simulink model "Input_Output"  (R2016b)
settings: Solver=FixedStepDiscrete  StartTime=0.0  StopTime=inf  FixedStep=InpOutp.tiSimnTiStep_C  RelTol=1e-3  EnableMultiTasking=on
settings Model: Creator=m01wolf  LastModifiedBy=bunver
settings DataIOCC: SaveFormat=StructureWithTime  SaveOutput=off  DSMLogging=off  VisualizeSimOutput=off  SaveTime=off  SignalLoggingName=Results
settings OptimizationCC: BlockReduction=off  ConditionallyExecuteInputs=off  LifeSpan=inf
settings DebuggingCC: AllowSymbolicDim=off  SFUnexpectedBacktrackingDiag=warning  SFNoUnconditionalDefaultTransitionDiag=warning  SFExecutionAtInitializationDiag=none
settings ModelReferenceCC: ModelReferenceNumInstancesAllowed=Single  PropagateSignalLabelsOutOfModel=off
settings GRTTargetCC: TargetLangStandard=C89/C90 (ANSI)
settings ConfigComp: CovMetricSettings=dw  CovHtmlReporting=on  CovSaveCumulativeToWorkspaceVar=on  CovSaveSingleToWorkspaceVar=on  CovExternalEMLEnable=off

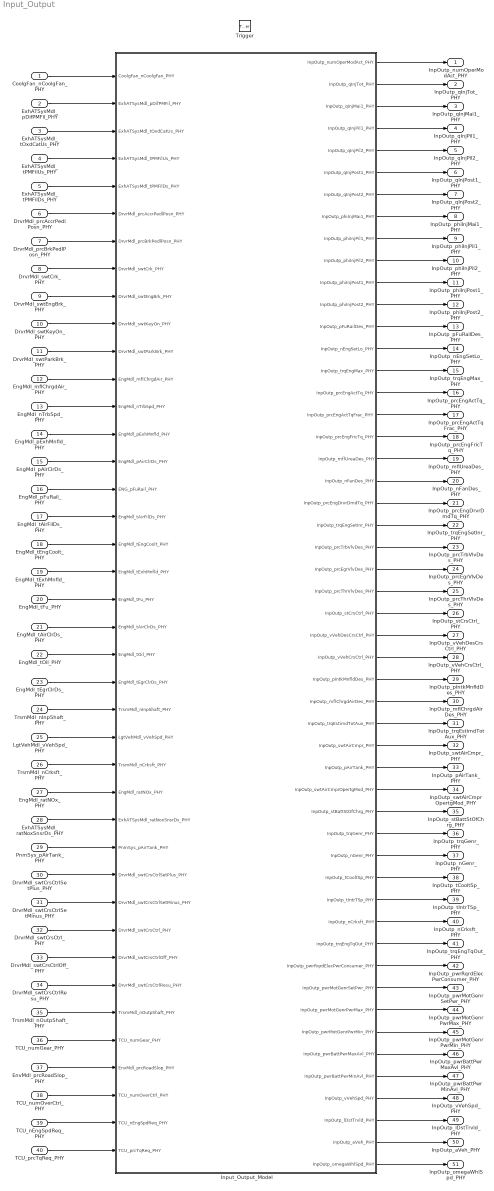
== system Input_Output ==
  CoolgFan_nCoolgFan_PHY : Inport
  ExhATSysMdl_pDifPMFil_PHY : Inport  Port=2
  ExhATSysMdl_tOxdCatUs_PHY : Inport  Port=3
  ExhATSysMdl_tPMFilUs_PHY : Inport  Port=4
  ExhATSysMdl_tPMFilDs_PHY : Inport  Port=5
  DrvrMdl_prcAccrPedlPosn_PHY : Inport  Port=6
  DrvrMdl_prcBrkPedlPosn_PHY : Inport  Port=7
  DrvrMdl_swtCrk_PHY : Inport  Port=8
  DrvrMdl_swtEngBrk_PHY : Inport  Port=9
  DrvrMdl_swtKeyOn_PHY : Inport  Port=10
  DrvrMdl_swtParkBrk_PHY : Inport  Port=11
  EngMdl_mflChrgdAir_PHY : Inport  Port=12
  EngMdl_nTrbSpd_PHY : Inport  Port=13
  EngMdl_pExhMnfld_PHY : Inport  Port=14
  EngMdl_pAirClrDs_PHY : Inport  Port=15
  EngMdl_pFuRail_PHY : Inport  Port=16
  EngMdl_tAirFilDs_PHY : Inport  Port=17
  EngMdl_tEngCoolt_PHY : Inport  Port=18
  EngMdl_tExhMnfld_PHY : Inport  Port=19
  EngMdl_tFu_PHY : Inport  Port=20
  EngMdl_tAirClrDs_PHY : Inport  Port=21
  EngMdl_tOil_PHY : Inport  Port=22
  EngMdl_tEgrClrDs_PHY : Inport  Port=23
  TrsmMdl_nInpShaft_PHY : Inport  Port=24
  LgtVehMdl_vVehSpd_PHY : Inport  Port=25
  TrsmMdl_nCrksft_PHY : Inport  Port=26
  EngMdl_ratNOx_PHY : Inport  Port=27
  ExhATSysMdl_ratNoxSnsrDs_PHY : Inport  Port=28
  PnmSys_pAirTank_PHY : Inport  Port=29
  DrvrMdl_swtCrsCtrlSetPlus_PHY : Inport  Port=30
  DrvrMdl_swtCrsCtrlSetMinus_PHY : Inport  Port=31
  DrvrMdl_swtCrsCtrl_PHY : Inport  Port=32
  DrvrMdl_swtCrsCtrlOff_PHY : Inport  Port=33
  DrvrMdl_swtCrsCtrlResu_PHY : Inport  Port=34
  TrsmMdl_nOutpShaft_PHY : Inport  Port=35
  TCU_numGear_PHY : Inport  Port=36
  EnvMdl_prcRoadSlop_PHY : Inport  Port=37
  TCU_numOverCtrl_PHY : Inport  Port=38
  TCU_nEngSpdReq_PHY : Inport  Port=39
  TCU_prcTqReq_PHY : Inport  Port=40
  Trigger : TriggerPort  TriggerType=function-call  VariantControl=Variant  PortDimensions=1
  Input_Output_Model : Subsystem
  InpOutp_numOperModAct_PHY : Outport
  InpOutp_qInjTot_PHY : Outport  Port=2
  InpOutp_qInjMai1_PHY : Outport  Port=3
  InpOutp_qInjPil1_PHY : Outport  Port=4
  InpOutp_qInjPil2_PHY : Outport  Port=5
  InpOutp_qInjPost1_PHY : Outport  Port=6
  InpOutp_qInjPost2_PHY : Outport  Port=7
  InpOutp_phiInjMai1_PHY : Outport  Port=8
  InpOutp_phiInjPil1_PHY : Outport  Port=9
  InpOutp_phiInjPil2_PHY : Outport  Port=10
  InpOutp_phiInjPost1_PHY : Outport  Port=11
  InpOutp_phiInjPost2_PHY : Outport  Port=12
  InpOutp_pFuRailDes_PHY : Outport  Port=13
  InpOutp_nEngSetLo_PHY : Outport  Port=14
  InpOutp_trqEngMax_PHY : Outport  Port=15
  InpOutp_prcEngActTq_PHY : Outport  Port=16
  InpOutp_prcEngActTqFrac_PHY : Outport  Port=17
  InpOutp_prcEngFricTq_PHY : Outport  Port=18
  InpOutp_mflUreaDes_PHY : Outport  Port=19
  InpOutp_nFanDes_PHY : Outport  Port=20
  InpOutp_prcEngDrvrDmdTq_PHY : Outport  Port=21
  InpOutp_trqEngSetInr_PHY : Outport  Port=22
  InpOutp_prcTrbVlvDes_PHY : Outport  Port=23
  InpOutp_prcEgrVlvDes_PHY : Outport  Port=24
  InpOutp_prcThrVlvDes_PHY : Outport  Port=25
  InpOutp_stCrsCtrl_PHY : Outport  Port=26
  InpOutp_vVehDesCrsCtrl_PHY : Outport  Port=27
  InpOutp_vVehCrsCtrl_PHY : Outport  Port=28
  InpOutp_pIntkMnfldDes_PHY : Outport  Port=29
  InpOutp_mflChrgdAirDes_PHY : Outport  Port=30
  InpOutp_trqEstimdTotAux_PHY : Outport  Port=31
  InpOutp_swtAirCmpr_PHY : Outport  Port=32
  InpOutp_pAirTank_PHY : Outport  Port=33
  InpOutp_swtAirCmprOpertgMod_PHY : Outport  Port=34
  InpOutp_stBattStOfChrg_PHY : Outport  Port=35
  InpOutp_trqGenr_PHY : Outport  Port=36
  InpOutp_nGenr_PHY : Outport  Port=37
  InpOutp_tCooltSp_PHY : Outport  Port=38
  InpOutp_tIntrTSp_PHY : Outport  Port=39
  InpOutp_nCrksft_PHY : Outport  Port=40
  InpOutp_trqEngTqOut_PHY : Outport  Port=41
  InpOutp_pwrRqrdElecPwrConsumer_PHY : Outport  Port=42
  InpOutp_pwrMotGenrSetPwr_PHY : Outport  Port=43
  InpOutp_pwrMotGenrPwrMax_PHY : Outport  Port=44
  InpOutp_pwrMotGenrPwrMin_PHY : Outport  Port=45
  InpOutp_pwrBattPwrMaxAvl_PHY : Outport  Port=46
  InpOutp_pwrBattPwrMinAvl_PHY : Outport  Port=47
  InpOutp_vVehSpd_PHY : Outport  Port=48
  InpOutp_lDstTrvld_PHY : Outport  Port=49
  InpOutp_aVeh_PHY : Outport  Port=50
  InpOutp_omegaWhlSpd_PHY : Outport  Port=51
  wires:
  Input_Output_Model/1(InpOutp_numOperModAct_PHY) -> InpOutp_numOperModAct_PHY/1
  Input_Output_Model/51(InpOutp_omegaWhlSpd_PHY) -> InpOutp_omegaWhlSpd_PHY/1
  Input_Output_Model/2(InpOutp_qInjTot_PHY) -> InpOutp_qInjTot_PHY/1
  Input_Output_Model/8(InpOutp_phiInjMai1_PHY) -> InpOutp_phiInjMai1_PHY/1
  Input_Output_Model/5(InpOutp_qInjPil2_PHY) -> InpOutp_qInjPil2_PHY/1
  Input_Output_Model/7(InpOutp_qInjPost2_PHY) -> InpOutp_qInjPost2_PHY/1
  Input_Output_Model/4(InpOutp_qInjPil1_PHY) -> InpOutp_qInjPil1_PHY/1
  Input_Output_Model/6(InpOutp_qInjPost1_PHY) -> InpOutp_qInjPost1_PHY/1
  Input_Output_Model/3(InpOutp_qInjMai1_PHY) -> InpOutp_qInjMai1_PHY/1
  Input_Output_Model/9(InpOutp_phiInjPil1_PHY) -> InpOutp_phiInjPil1_PHY/1
  Input_Output_Model/10(InpOutp_phiInjPil2_PHY) -> InpOutp_phiInjPil2_PHY/1
  Input_Output_Model/11(InpOutp_phiInjPost1_PHY) -> InpOutp_phiInjPost1_PHY/1
  Input_Output_Model/12(InpOutp_phiInjPost2_PHY) -> InpOutp_phiInjPost2_PHY/1
  Input_Output_Model/13(InpOutp_pFuRailDes_PHY) -> InpOutp_pFuRailDes_PHY/1
  Input_Output_Model/14(InpOutp_nEngSetLo_PHY) -> InpOutp_nEngSetLo_PHY/1
  Input_Output_Model/15(InpOutp_trqEngMax_PHY) -> InpOutp_trqEngMax_PHY/1
  Input_Output_Model/16(InpOutp_prcEngActTq_PHY) -> InpOutp_prcEngActTq_PHY/1
  Input_Output_Model/17(InpOutp_prcEngActTqFrac_PHY) -> InpOutp_prcEngActTqFrac_PHY/1
  Input_Output_Model/18(InpOutp_prcEngFricTq_PHY) -> InpOutp_prcEngFricTq_PHY/1
  Input_Output_Model/19(InpOutp_mflUreaDes_PHY) -> InpOutp_mflUreaDes_PHY/1
  Input_Output_Model/20(InpOutp_nFanDes_PHY) -> InpOutp_nFanDes_PHY/1
  Input_Output_Model/21(InpOutp_prcEngDrvrDmdTq_PHY) -> InpOutp_prcEngDrvrDmdTq_PHY/1
  Input_Output_Model/22(InpOutp_trqEngSetInr_PHY) -> InpOutp_trqEngSetInr_PHY/1
  Input_Output_Model/23(InpOutp_prcTrbVlvDes_PHY) -> InpOutp_prcTrbVlvDes_PHY/1
  Input_Output_Model/24(InpOutp_prcEgrVlvDes_PHY) -> InpOutp_prcEgrVlvDes_PHY/1
  Input_Output_Model/25(InpOutp_prcThrVlvDes_PHY) -> InpOutp_prcThrVlvDes_PHY/1
  Input_Output_Model/26(InpOutp_stCrsCtrl_PHY) -> InpOutp_stCrsCtrl_PHY/1
  Input_Output_Model/27(InpOutp_vVehDesCrsCtrl_PHY) -> InpOutp_vVehDesCrsCtrl_PHY/1
  Input_Output_Model/28(InpOutp_vVehCrsCtrl_PHY) -> InpOutp_vVehCrsCtrl_PHY/1
  Input_Output_Model/29(InpOutp_pIntkMnfldDes_PHY) -> InpOutp_pIntkMnfldDes_PHY/1
  Input_Output_Model/30(InpOutp_mflChrgdAirDes_PHY) -> InpOutp_mflChrgdAirDes_PHY/1
  Input_Output_Model/31(InpOutp_trqEstimdTotAux_PHY) -> InpOutp_trqEstimdTotAux_PHY/1
  Input_Output_Model/32(InpOutp_swtAirCmpr_PHY) -> InpOutp_swtAirCmpr_PHY/1
  Input_Output_Model/33(InpOutp_pAirTank_PHY) -> InpOutp_pAirTank_PHY/1
  Input_Output_Model/34(InpOutp_swtAirCmprOpertgMod_PHY) -> InpOutp_swtAirCmprOpertgMod_PHY/1
  Input_Output_Model/35(InpOutp_stBattStOfChrg_PHY) -> InpOutp_stBattStOfChrg_PHY/1
  Input_Output_Model/36(InpOutp_trqGenr_PHY) -> InpOutp_trqGenr_PHY/1
  Input_Output_Model/37(InpOutp_nGenr_PHY) -> InpOutp_nGenr_PHY/1
  Input_Output_Model/38(InpOutp_tCooltSp_PHY) -> InpOutp_tCooltSp_PHY/1
  Input_Output_Model/39(InpOutp_tIntrTSp_PHY) -> InpOutp_tIntrTSp_PHY/1
  Input_Output_Model/40(InpOutp_nCrksft_PHY) -> InpOutp_nCrksft_PHY/1
  Input_Output_Model/41(InpOutp_trqEngTqOut_PHY) -> InpOutp_trqEngTqOut_PHY/1
  Input_Output_Model/42(InpOutp_pwrRqrdElecPwrConsumer_PHY) -> InpOutp_pwrRqrdElecPwrConsumer_PHY/1
  Input_Output_Model/43(InpOutp_pwrMotGenrSetPwr_PHY) -> InpOutp_pwrMotGenrSetPwr_PHY/1
  Input_Output_Model/44(InpOutp_pwrMotGenrPwrMax_PHY) -> InpOutp_pwrMotGenrPwrMax_PHY/1
  Input_Output_Model/45(InpOutp_pwrMotGenrPwrMin_PHY) -> InpOutp_pwrMotGenrPwrMin_PHY/1
  Input_Output_Model/46(InpOutp_pwrBattPwrMaxAvl_PHY) -> InpOutp_pwrBattPwrMaxAvl_PHY/1
  Input_Output_Model/47(InpOutp_pwrBattPwrMinAvl_PHY) -> InpOutp_pwrBattPwrMinAvl_PHY/1
  Input_Output_Model/48(InpOutp_vVehSpd_PHY) -> InpOutp_vVehSpd_PHY/1
  Input_Output_Model/49(InpOutp_lDstTrvld_PHY) -> InpOutp_lDstTrvld_PHY/1
  Input_Output_Model/50(InpOutp_aVeh_PHY) -> InpOutp_aVeh_PHY/1
  CoolgFan_nCoolgFan_PHY/1 -> Input_Output_Model/1(CoolgFan_nCoolgFan_PHY)
  TCU_prcTqReq_PHY/1 -> Input_Output_Model/40(TCU_prcTqReq_PHY)
  ExhATSysMdl_pDifPMFil_PHY/1 -> Input_Output_Model/2(ExhATSysMdl_pDifPMFil_PHY)
  ExhATSysMdl_tOxdCatUs_PHY/1 -> Input_Output_Model/3(ExhATSysMdl_tOxdCatUs_PHY)
  ExhATSysMdl_tPMFilUs_PHY/1 -> Input_Output_Model/4(ExhATSysMdl_tPMFilUs_PHY)
  ExhATSysMdl_tPMFilDs_PHY/1 -> Input_Output_Model/5(ExhATSysMdl_tPMFilDs_PHY)
  DrvrMdl_prcAccrPedlPosn_PHY/1 -> Input_Output_Model/6(DrvrMdl_prcAccrPedlPosn_PHY)
  DrvrMdl_prcBrkPedlPosn_PHY/1 -> Input_Output_Model/7(DrvrMdl_prcBrkPedlPosn_PHY)
  DrvrMdl_swtCrk_PHY/1 -> Input_Output_Model/8(DrvrMdl_swtCrk_PHY)
  DrvrMdl_swtEngBrk_PHY/1 -> Input_Output_Model/9(DrvrMdl_swtEngBrk_PHY)
  DrvrMdl_swtKeyOn_PHY/1 -> Input_Output_Model/10(DrvrMdl_swtKeyOn_PHY)
  DrvrMdl_swtParkBrk_PHY/1 -> Input_Output_Model/11(DrvrMdl_swtParkBrk_PHY)
  EngMdl_mflChrgdAir_PHY/1 -> Input_Output_Model/12(EngMdl_mflChrgdAir_PHY)
  EngMdl_nTrbSpd_PHY/1 -> Input_Output_Model/13(EngMdl_nTrbSpd_PHY)
  EngMdl_pExhMnfld_PHY/1 -> Input_Output_Model/14(EngMdl_pExhMnfld_PHY)
  EngMdl_pAirClrDs_PHY/1 -> Input_Output_Model/15(EngMdl_pAirClrDs_PHY)
  EngMdl_pFuRail_PHY/1 -> Input_Output_Model/16(ENG_pFuRail_PHY)
  EngMdl_tAirFilDs_PHY/1 -> Input_Output_Model/17(EngMdl_tAirFilDs_PHY)
  EngMdl_tEngCoolt_PHY/1 -> Input_Output_Model/18(EngMdl_tEngCoolt_PHY)
  EngMdl_tExhMnfld_PHY/1 -> Input_Output_Model/19(EngMdl_tExhMnfld_PHY)
  EngMdl_tFu_PHY/1 -> Input_Output_Model/20(EngMdl_tFu_PHY)
  EngMdl_tAirClrDs_PHY/1 -> Input_Output_Model/21(EngMdl_tAirClrDs_PHY)
  EngMdl_tOil_PHY/1 -> Input_Output_Model/22(EngMdl_tOil_PHY)
  EngMdl_tEgrClrDs_PHY/1 -> Input_Output_Model/23(EngMdl_tEgrClrDs_PHY)
  TrsmMdl_nInpShaft_PHY/1 -> Input_Output_Model/24(TrsmMdl_nInpShaft_PHY)
  LgtVehMdl_vVehSpd_PHY/1 -> Input_Output_Model/25(LgtVehMdl_vVehSpd_PHY)
  TrsmMdl_nCrksft_PHY/1 -> Input_Output_Model/26(TrsmMdl_nCrksft_PHY)
  EngMdl_ratNOx_PHY/1 -> Input_Output_Model/27(EngMdl_ratNOx_PHY)
  ExhATSysMdl_ratNoxSnsrDs_PHY/1 -> Input_Output_Model/28(ExhATSysMdl_ratNoxSnsrDs_PHY)
  PnmSys_pAirTank_PHY/1 -> Input_Output_Model/29(PnmSys_pAirTank_PHY)
  DrvrMdl_swtCrsCtrlSetPlus_PHY/1 -> Input_Output_Model/30(DrvrMdl_swtCrsCtrlSetPlus_PHY)
  DrvrMdl_swtCrsCtrlSetMinus_PHY/1 -> Input_Output_Model/31(DrvrMdl_swtCrsCtrlSetMinus_PHY)
  DrvrMdl_swtCrsCtrl_PHY/1 -> Input_Output_Model/32(DrvrMdl_swtCrsCtrl_PHY)
  DrvrMdl_swtCrsCtrlOff_PHY/1 -> Input_Output_Model/33(DrvrMdl_swtCrsCtrlOff_PHY)
  DrvrMdl_swtCrsCtrlResu_PHY/1 -> Input_Output_Model/34(DrvrMdl_swtCrsCtrlResu_PHY)
  TrsmMdl_nOutpShaft_PHY/1 -> Input_Output_Model/35(TrsmMdl_nOutpShaft_PHY)
  TCU_numGear_PHY/1 -> Input_Output_Model/36(TCU_numGear_PHY)
  EnvMdl_prcRoadSlop_PHY/1 -> Input_Output_Model/37(EnvMdl_prcRoadSlop_PHY)
  TCU_numOverCtrl_PHY/1 -> Input_Output_Model/38(TCU_numOverCtrl_PHY)
  TCU_nEngSpdReq_PHY/1 -> Input_Output_Model/39(TCU_nEngSpdReq_PHY)

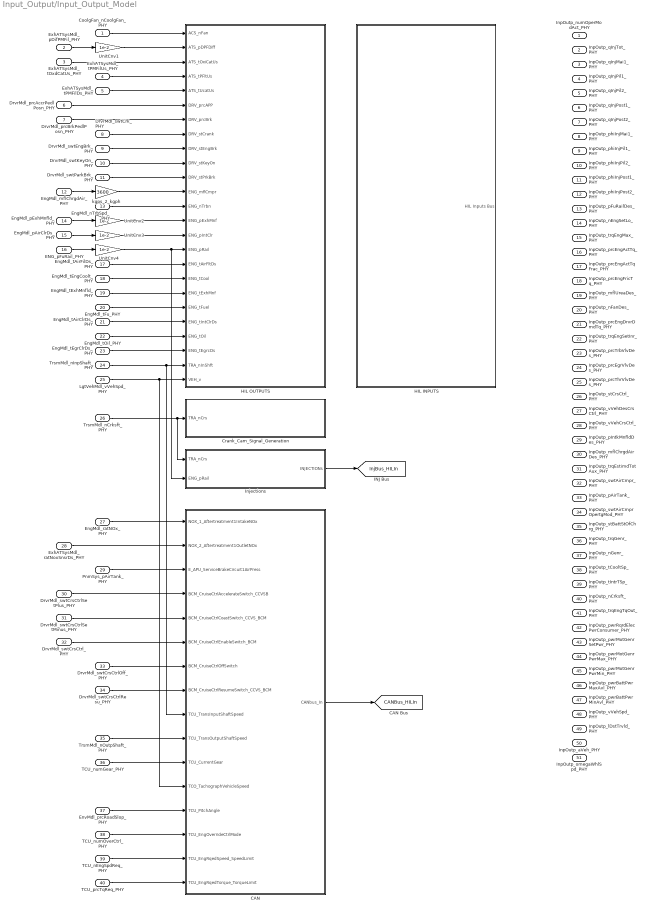
== system Input_Output/Input_Output_Model ==
  CoolgFan_nCoolgFan_PHY : Inport
  ExhATSysMdl_pDifPMFil_PHY : Inport  Port=2
  ExhATSysMdl_tOxdCatUs_PHY : Inport  Port=3
  ExhATSysMdl_tPMFilUs_PHY : Inport  Port=4
  ExhATSysMdl_tPMFilDs_PHY : Inport  Port=5
  DrvrMdl_prcAccrPedlPosn_PHY : Inport  Port=6
  DrvrMdl_prcBrkPedlPosn_PHY : Inport  Port=7
  DrvrMdl_swtCrk_PHY : Inport  Port=8
  DrvrMdl_swtEngBrk_PHY : Inport  Port=9
  DrvrMdl_swtKeyOn_PHY : Inport  Port=10
  DrvrMdl_swtParkBrk_PHY : Inport  Port=11
  EngMdl_mflChrgdAir_PHY : Inport  Port=12
  EngMdl_nTrbSpd_PHY : Inport  Port=13
  EngMdl_pExhMnfld_PHY : Inport  Port=14
  EngMdl_pAirClrDs_PHY : Inport  Port=15
  ENG_pFuRail_PHY : Inport  Port=16
  EngMdl_tAirFilDs_PHY : Inport  Port=17
  EngMdl_tEngCoolt_PHY : Inport  Port=18
  EngMdl_tExhMnfld_PHY : Inport  Port=19
  EngMdl_tFu_PHY : Inport  Port=20
  EngMdl_tAirClrDs_PHY : Inport  Port=21
  EngMdl_tOil_PHY : Inport  Port=22
  EngMdl_tEgrClrDs_PHY : Inport  Port=23
  TrsmMdl_nInpShaft_PHY : Inport  Port=24
  LgtVehMdl_vVehSpd_PHY : Inport  Port=25
  TrsmMdl_nCrksft_PHY : Inport  Port=26
  EngMdl_ratNOx_PHY : Inport  Port=27
  ExhATSysMdl_ratNoxSnsrDs_PHY : Inport  Port=28
  PnmSys_pAirTank_PHY : Inport  Port=29
  DrvrMdl_swtCrsCtrlSetPlus_PHY : Inport  Port=30
  DrvrMdl_swtCrsCtrlSetMinus_PHY : Inport  Port=31
  DrvrMdl_swtCrsCtrl_PHY : Inport  Port=32
  DrvrMdl_swtCrsCtrlOff_PHY : Inport  Port=33
  DrvrMdl_swtCrsCtrlResu_PHY : Inport  Port=34
  TrsmMdl_nOutpShaft_PHY : Inport  Port=35
  TCU_numGear_PHY : Inport  Port=36
  EnvMdl_prcRoadSlop_PHY : Inport  Port=37
  TCU_numOverCtrl_PHY : Inport  Port=38
  TCU_nEngSpdReq_PHY : Inport  Port=39
  TCU_prcTqReq_PHY : Inport  Port=40
  CAN : Subsystem
  Crank_Cam_Signal_Generation : Subsystem
  HIL INPUTS : Subsystem
  HIL OUTPUTS : Subsystem
  Injections : Subsystem
  UnitCnv{1..4} (4 alike) : Gain  Gain=1e-2  SaturateOnIntegerOverflow=on  OutDataTypeStr=Inherit: Same as input  ParamDataTypeStr=Inherit: Same as input
  kgps_2_kgph : Gain  Gain=3600
  InpOutp_numOperModAct_PHY : Outport
  InpOutp_qInjTot_PHY : Outport  Port=2
  InpOutp_qInjMai1_PHY : Outport  Port=3
  InpOutp_qInjPil1_PHY : Outport  Port=4
  InpOutp_qInjPil2_PHY : Outport  Port=5
  InpOutp_qInjPost1_PHY : Outport  Port=6
  InpOutp_qInjPost2_PHY : Outport  Port=7
  InpOutp_phiInjMai1_PHY : Outport  Port=8
  InpOutp_phiInjPil1_PHY : Outport  Port=9
  InpOutp_phiInjPil2_PHY : Outport  Port=10
  InpOutp_phiInjPost1_PHY : Outport  Port=11
  InpOutp_phiInjPost2_PHY : Outport  Port=12
  InpOutp_pFuRailDes_PHY : Outport  Port=13
  InpOutp_nEngSetLo_PHY : Outport  Port=14
  InpOutp_trqEngMax_PHY : Outport  Port=15
  InpOutp_prcEngActTq_PHY : Outport  Port=16
  InpOutp_prcEngActTqFrac_PHY : Outport  Port=17
  InpOutp_prcEngFricTq_PHY : Outport  Port=18
  InpOutp_mflUreaDes_PHY : Outport  Port=19
  InpOutp_nFanDes_PHY : Outport  Port=20
  InpOutp_prcEngDrvrDmdTq_PHY : Outport  Port=21
  InpOutp_trqEngSetInr_PHY : Outport  Port=22
  InpOutp_prcTrbVlvDes_PHY : Outport  Port=23
  InpOutp_prcEgrVlvDes_PHY : Outport  Port=24
  InpOutp_prcThrVlvDes_PHY : Outport  Port=25
  InpOutp_stCrsCtrl_PHY : Outport  Port=26
  InpOutp_vVehDesCrsCtrl_PHY : Outport  Port=27
  InpOutp_vVehCrsCtrl_PHY : Outport  Port=28
  InpOutp_pIntkMnfldDes_PHY : Outport  Port=29
  InpOutp_mflChrgdAirDes_PHY : Outport  Port=30
  InpOutp_trqEstimdTotAux_PHY : Outport  Port=31
  InpOutp_swtAirCmpr_PHY : Outport  Port=32
  InpOutp_pAirTank_PHY : Outport  Port=33
  InpOutp_swtAirCmprOpertgMod_PHY : Outport  Port=34
  InpOutp_stBattStOfChrg_PHY : Outport  Port=35
  InpOutp_trqGenr_PHY : Outport  Port=36
  InpOutp_nGenr_PHY : Outport  Port=37
  InpOutp_tCooltSp_PHY : Outport  Port=38
  InpOutp_tIntrTSp_PHY : Outport  Port=39
  InpOutp_nCrksft_PHY : Outport  Port=40
  InpOutp_trqEngTqOut_PHY : Outport  Port=41
  InpOutp_pwrRqrdElecPwrConsumer_PHY : Outport  Port=42
  InpOutp_pwrMotGenrSetPwr_PHY : Outport  Port=43
  InpOutp_pwrMotGenrPwrMax_PHY : Outport  Port=44
  InpOutp_pwrMotGenrPwrMin_PHY : Outport  Port=45
  InpOutp_pwrBattPwrMaxAvl_PHY : Outport  Port=46
  InpOutp_pwrBattPwrMinAvl_PHY : Outport  Port=47
  InpOutp_vVehSpd_PHY : Outport  Port=48
  InpOutp_lDstTrvld_PHY : Outport  Port=49
  InpOutp_aVeh_PHY : Outport  Port=50
  InpOutp_omegaWhlSpd_PHY : Outport  Port=51
  tag scope: CANBus_HILIn=global, InjBus_HILIn=global
  wires:
  Injections/1(INJECTIONs) -> [InjBus_HILIn]
  TrsmMdl_nCrksft_PHY/1 -> Injections/1(TRA_nCrs), Crank_Cam_Signal_Generation/1(TRA_nCrs)
  UnitCnv4/1 -> Injections/2(ENG_pRail), HIL OUTPUTS/16(ENG_pRail)
  CoolgFan_nCoolgFan_PHY/1 -> HIL OUTPUTS/1(ACS_nFan)
  ExhATSysMdl_pDifPMFil_PHY/1 -> UnitCnv1/1
  ExhATSysMdl_tOxdCatUs_PHY/1 -> HIL OUTPUTS/3(ATS_tOxiCatUs)
  ExhATSysMdl_tPMFilUs_PHY/1 -> HIL OUTPUTS/4(ATS_tPFltUs)
  DrvrMdl_prcAccrPedlPosn_PHY/1 -> HIL OUTPUTS/6(DRV_prcAPP)
  DrvrMdl_prcBrkPedlPosn_PHY/1 -> HIL OUTPUTS/7(DRV_prcBrk)
  ExhATSysMdl_tPMFilDs_PHY/1 -> HIL OUTPUTS/5(ATS_tUcatUs)
  DrvrMdl_swtEngBrk_PHY/1 -> HIL OUTPUTS/9(DRV_stEngBrk)
  DrvrMdl_swtCrk_PHY/1 -> HIL OUTPUTS/8(DRV_stCrank)
  DrvrMdl_swtKeyOn_PHY/1 -> HIL OUTPUTS/10(DRV_stKeyOn)
  EngMdl_pAirClrDs_PHY/1 -> UnitCnv3/1
  EngMdl_pExhMnfld_PHY/1 -> UnitCnv2/1
  DrvrMdl_swtParkBrk_PHY/1 -> HIL OUTPUTS/11(DRV_stPrkBrk)
  EngMdl_nTrbSpd_PHY/1 -> HIL OUTPUTS/13(ENG_nTrbn)
  EngMdl_mflChrgdAir_PHY/1 -> kgps_2_kgph/1
  ENG_pFuRail_PHY/1 -> UnitCnv4/1
  EngMdl_tFu_PHY/1 -> HIL OUTPUTS/20(ENG_tFuel)
  EngMdl_tExhMnfld_PHY/1 -> HIL OUTPUTS/19(ENG_tExhMnf)
  EngMdl_tAirFilDs_PHY/1 -> HIL OUTPUTS/17(ENG_tAirFltDs)
  EngMdl_tEngCoolt_PHY/1 -> HIL OUTPUTS/18(ENG_tCool)
  EngMdl_tAirClrDs_PHY/1 -> HIL OUTPUTS/21(ENG_tIntClrDs)
  EngMdl_tEgrClrDs_PHY/1 -> HIL OUTPUTS/23(ENG_tEgrcDs)
  EngMdl_tOil_PHY/1 -> HIL OUTPUTS/22(ENG_tOil)
  TrsmMdl_nInpShaft_PHY/1 -> CAN/9(TCU_TransInputShaftSpeed), HIL OUTPUTS/24(TRA_nInShft)
  LgtVehMdl_vVehSpd_PHY/1 -> CAN/12(TCO_TachographVehicleSpeed), HIL OUTPUTS/25(VEH_v)
  UnitCnv1/1 -> HIL OUTPUTS/2(ATS_pDPFDiff)
  kgps_2_kgph/1 -> HIL OUTPUTS/12(ENG_mflCmpr)
  UnitCnv2/1 -> HIL OUTPUTS/14(ENG_pExhMnf)
  UnitCnv3/1 -> HIL OUTPUTS/15(ENG_pIntClr)
  EngMdl_ratNOx_PHY/1 -> CAN/1(NOX_1_Aftertreatment1IntakeNOx)
  ExhATSysMdl_ratNoxSnsrDs_PHY/1 -> CAN/2(NOX_2_Aftertreatment1OutletNOx)
  PnmSys_pAirTank_PHY/1 -> CAN/3(E_APU_ServiceBrakeCircuit1AirPress)
  DrvrMdl_swtCrsCtrlSetPlus_PHY/1 -> CAN/4(BCM_CruiseCtrlAccelerateSwitch_CCVSB)
  DrvrMdl_swtCrsCtrlSetMinus_PHY/1 -> CAN/5(BCM_CruiseCtrlCoastSwitch_CCVS_BCM)
  DrvrMdl_swtCrsCtrl_PHY/1 -> CAN/6(BCM_CruiseCtrlEnableSwitch_BCM)
  DrvrMdl_swtCrsCtrlOff_PHY/1 -> CAN/7(BCM_CruiseCtrlOffSwitch)
  DrvrMdl_swtCrsCtrlResu_PHY/1 -> CAN/8(BCM_CruiseCtrlResumeSwitch_CCVS_BCM)
  TrsmMdl_nOutpShaft_PHY/1 -> CAN/10(TCU_TransOutputShaftSpeed)
  TCU_numGear_PHY/1 -> CAN/11(TCU_CurrentGear)
  EnvMdl_prcRoadSlop_PHY/1 -> CAN/13(TCU_PitchAngle)
  TCU_numOverCtrl_PHY/1 -> CAN/14(TCU_EngOverrideCtrlMode)
  TCU_nEngSpdReq_PHY/1 -> CAN/15(TCU_EngRqedSpeed_SpeedLimit)
  TCU_prcTqReq_PHY/1 -> CAN/16(TCU_EngRqedTorque_TorqueLimit)
  CAN/1(CANbus_In) -> [CANBus_HILIn]

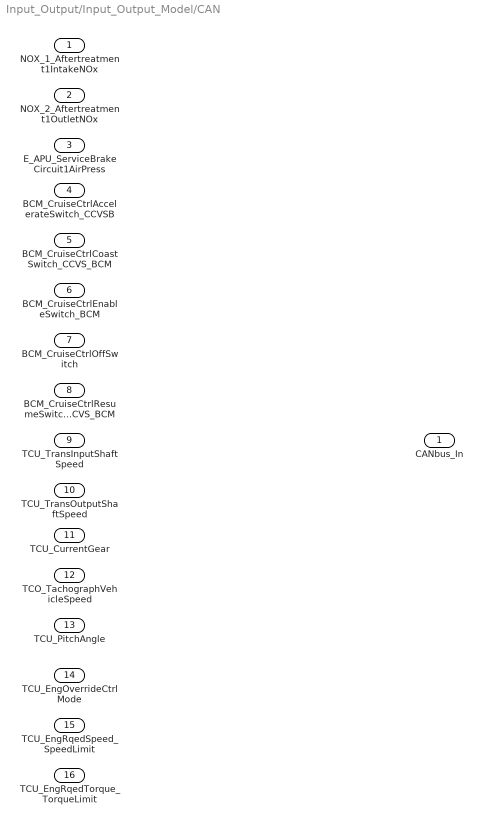
== system Input_Output/Input_Output_Model/CAN ==
  NOX_1_Aftertreatment1IntakeNOx : Inport
  NOX_2_Aftertreatment1OutletNOx : Inport  Port=2
  E_APU_ServiceBrakeCircuit1AirPress : Inport  Port=3
  BCM_CruiseCtrlAccelerateSwitch_CCVSB : Inport  Port=4
  BCM_CruiseCtrlCoastSwitch_CCVS_BCM : Inport  Port=5
  BCM_CruiseCtrlEnableSwitch_BCM : Inport  Port=6
  BCM_CruiseCtrlOffSwitch : Inport  Port=7
  BCM_CruiseCtrlResumeSwitch_CCVS_BCM : Inport  Port=8
  TCU_TransInputShaftSpeed : Inport  Port=9
  TCU_TransOutputShaftSpeed : Inport  Port=10
  TCU_CurrentGear : Inport  Port=11
  TCO_TachographVehicleSpeed : Inport  Port=12
  TCU_PitchAngle : Inport  Port=13
  TCU_EngOverrideCtrlMode : Inport  Port=14
  TCU_EngRqedSpeed_SpeedLimit : Inport  Port=15
  TCU_EngRqedTorque_TorqueLimit : Inport  Port=16
  CANbus_In : Outport

== system Input_Output/Input_Output_Model/Crank_Cam_Signal_Generation ==
  TRA_nCrs : Inport
  Terminator : Terminator
  wires:
  TRA_nCrs/1 -> Terminator/1

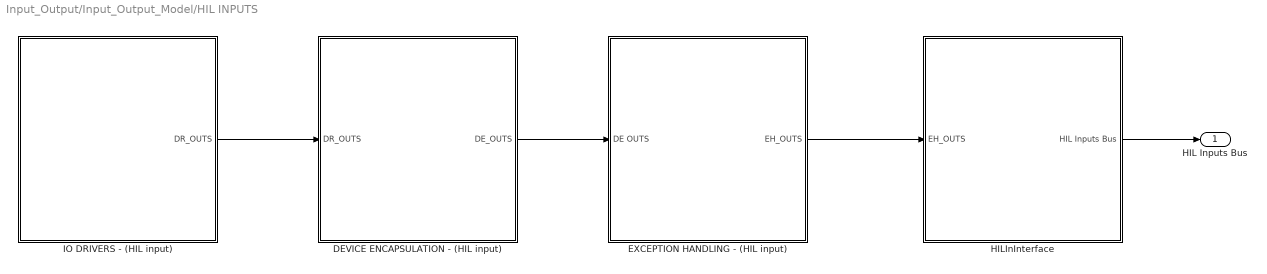
== system Input_Output/Input_Output_Model/HIL INPUTS ==
  DEVICE ENCAPSULATION - (HIL input) : Subsystem
  EXCEPTION HANDLING - (HIL input) : Subsystem
  HILInInterface : Subsystem
  IO DRIVERS - (HIL input) : Subsystem
  HIL Inputs Bus : Outport
  wires:
  HILInInterface/1(HIL Inputs Bus) -> HIL Inputs Bus/1
  EXCEPTION HANDLING - (HIL input)/1(EH_OUTS) -> HILInInterface/1(EH_OUTS)
  DEVICE ENCAPSULATION - (HIL input)/1(DE_OUTS) -> EXCEPTION HANDLING - (HIL input)/1(DE OUTS)
  IO DRIVERS - (HIL input)/1(DR_OUTS) -> DEVICE ENCAPSULATION - (HIL input)/1(DR_OUTS)

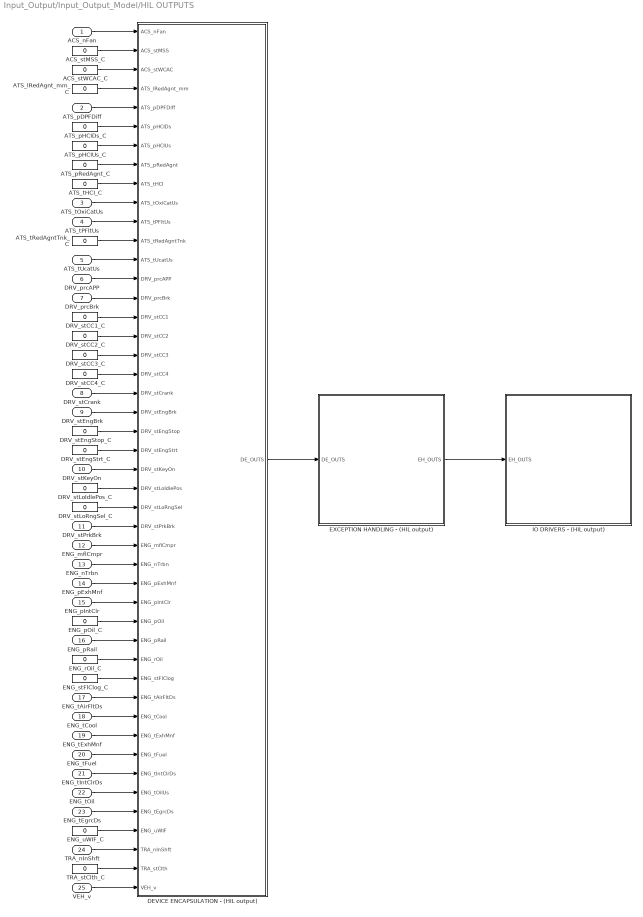
== system Input_Output/Input_Output_Model/HIL OUTPUTS ==
  ACS_nFan : Inport
  ATS_pDPFDiff : Inport  Port=2
  ATS_tOxiCatUs : Inport  Port=3
  ATS_tPFltUs : Inport  Port=4
  ATS_tUcatUs : Inport  Port=5
  DRV_prcAPP : Inport  Port=6
  DRV_prcBrk : Inport  Port=7
  DRV_stCrank : Inport  Port=8
  DRV_stEngBrk : Inport  Port=9
  DRV_stKeyOn : Inport  Port=10
  DRV_stPrkBrk : Inport  Port=11
  ENG_mflCmpr : Inport  Port=12
  ENG_nTrbn : Inport  Port=13
  ENG_pExhMnf : Inport  Port=14
  ENG_pIntClr : Inport  Port=15
  ENG_pRail : Inport  Port=16
  ENG_tAirFltDs : Inport  Port=17
  ENG_tCool : Inport  Port=18
  ENG_tExhMnf : Inport  Port=19
  ENG_tFuel : Inport  Port=20
  ENG_tIntClrDs : Inport  Port=21
  ENG_tOil : Inport  Port=22
  ENG_tEgrcDs : Inport  Port=23
  TRA_nInShft : Inport  Port=24
  VEH_v : Inport  Port=25
  ACS_stMSS_C : Constant  Value=0
  ACS_stWCAC_C : Constant  Value=0
  ATS_lRedAgnt_mm_C : Constant  Value=0
  ATS_pHCIDs_C : Constant  Value=0
  ATS_pHCIUs_C : Constant  Value=0
  ATS_pRedAgnt_C : Constant  Value=0
  ATS_tHCI_C : Constant  Value=0
  ATS_tRedAgntTnk_C : Constant  Value=0
  DEVICE ENCAPSULATION - (HIL output) : Subsystem
  DRV_stCC1_C : Constant  Value=0
  DRV_stCC2_C : Constant  Value=0
  DRV_stCC3_C : Constant  Value=0
  DRV_stCC4_C : Constant  Value=0
  DRV_stEngStop_C : Constant  Value=0
  DRV_stEngStrt_C : Constant  Value=0
  DRV_stLoIdlePos_C : Constant  Value=0
  DRV_stLoRngSel_C : Constant  Value=0
  ENG_pOil_C : Constant  Value=0
  ENG_rOil_C : Constant  Value=0
  ENG_stFlClog_C : Constant  Value=0
  ENG_uWIF_C : Constant  Value=0
  EXCEPTION HANDLING - (HIL output) : Subsystem
  IO DRIVERS - (HIL output) : Subsystem
  TRA_stClth_C : Constant  Value=0
  wires:
  EXCEPTION HANDLING - (HIL output)/1(EH_OUTS) -> IO DRIVERS - (HIL output)/1(EH_OUTS)
  DEVICE ENCAPSULATION - (HIL output)/1(DE_OUTS) -> EXCEPTION HANDLING - (HIL output)/1(DE_OUTS)
  ACS_nFan/1 -> DEVICE ENCAPSULATION - (HIL output)/1(ACS_nFan)
  ENG_mflCmpr/1 -> DEVICE ENCAPSULATION - (HIL output)/28(ENG_mflCmpr)
  VEH_v/1 -> DEVICE ENCAPSULATION - (HIL output)/46(VEH_v)
  TRA_nInShft/1 -> DEVICE ENCAPSULATION - (HIL output)/44(TRA_nInShft)
  ENG_nTrbn/1 -> DEVICE ENCAPSULATION - (HIL output)/29(ENG_nTrbn)
  ATS_pDPFDiff/1 -> DEVICE ENCAPSULATION - (HIL output)/5(ATS_pDPFDiff)
  ENG_pExhMnf/1 -> DEVICE ENCAPSULATION - (HIL output)/30(ENG_pExhMnf)
  DRV_prcAPP/1 -> DEVICE ENCAPSULATION - (HIL output)/14(DRV_prcAPP)
  ENG_pRail/1 -> DEVICE ENCAPSULATION - (HIL output)/33(ENG_pRail)
  ENG_pIntClr/1 -> DEVICE ENCAPSULATION - (HIL output)/31(ENG_pIntClr)
  ATS_tOxiCatUs/1 -> DEVICE ENCAPSULATION - (HIL output)/10(ATS_tOxiCatUs)
  ATS_tPFltUs/1 -> DEVICE ENCAPSULATION - (HIL output)/11(ATS_tPFltUs)
  ENG_tExhMnf/1 -> DEVICE ENCAPSULATION - (HIL output)/38(ENG_tExhMnf)
  ENG_tFuel/1 -> DEVICE ENCAPSULATION - (HIL output)/39(ENG_tFuel)
  ENG_tCool/1 -> DEVICE ENCAPSULATION - (HIL output)/37(ENG_tCool)
  ENG_tAirFltDs/1 -> DEVICE ENCAPSULATION - (HIL output)/36(ENG_tAirFltDs)
  ENG_tIntClrDs/1 -> DEVICE ENCAPSULATION - (HIL output)/40(ENG_tIntClrDs)
  ENG_tEgrcDs/1 -> DEVICE ENCAPSULATION - (HIL output)/42(ENG_tEgrcDs)
  ENG_tOil/1 -> DEVICE ENCAPSULATION - (HIL output)/41(ENG_tOilUs)
  ATS_tUcatUs/1 -> DEVICE ENCAPSULATION - (HIL output)/13(ATS_tUcatUs)
  TRA_stClth_C/1 -> DEVICE ENCAPSULATION - (HIL output)/45(TRA_stClth)
  DRV_prcBrk/1 -> DEVICE ENCAPSULATION - (HIL output)/15(DRV_prcBrk)
  DRV_stEngBrk/1 -> DEVICE ENCAPSULATION - (HIL output)/21(DRV_stEngBrk)
  DRV_stPrkBrk/1 -> DEVICE ENCAPSULATION - (HIL output)/27(DRV_stPrkBrk)
  DRV_stKeyOn/1 -> DEVICE ENCAPSULATION - (HIL output)/24(DRV_stKeyOn)
  DRV_stCrank/1 -> DEVICE ENCAPSULATION - (HIL output)/20(DRV_stCrank)
  ACS_stMSS_C/1 -> DEVICE ENCAPSULATION - (HIL output)/2(ACS_stMSS)
  DRV_stCC1_C/1 -> DEVICE ENCAPSULATION - (HIL output)/16(DRV_stCC1)
  DRV_stCC2_C/1 -> DEVICE ENCAPSULATION - (HIL output)/17(DRV_stCC2)
  DRV_stCC3_C/1 -> DEVICE ENCAPSULATION - (HIL output)/18(DRV_stCC3)
  DRV_stCC4_C/1 -> DEVICE ENCAPSULATION - (HIL output)/19(DRV_stCC4)
  ACS_stWCAC_C/1 -> DEVICE ENCAPSULATION - (HIL output)/3(ACS_stWCAC)
  DRV_stEngStop_C/1 -> DEVICE ENCAPSULATION - (HIL output)/22(DRV_stEngStop)
  DRV_stEngStrt_C/1 -> DEVICE ENCAPSULATION - (HIL output)/23(DRV_stEngStrt)
  ENG_stFlClog_C/1 -> DEVICE ENCAPSULATION - (HIL output)/35(ENG_stFlClog)
  ENG_uWIF_C/1 -> DEVICE ENCAPSULATION - (HIL output)/43(ENG_uWIF)
  DRV_stLoIdlePos_C/1 -> DEVICE ENCAPSULATION - (HIL output)/25(DRV_stLoIdlePos)
  DRV_stLoRngSel_C/1 -> DEVICE ENCAPSULATION - (HIL output)/26(DRV_stLoRngSel)
  ENG_pOil_C/1 -> DEVICE ENCAPSULATION - (HIL output)/32(ENG_pOil)
  ENG_rOil_C/1 -> DEVICE ENCAPSULATION - (HIL output)/34(ENG_rOil)
  ATS_lRedAgnt_mm_C/1 -> DEVICE ENCAPSULATION - (HIL output)/4(ATS_lRedAgnt_mm)
  ATS_pHCIDs_C/1 -> DEVICE ENCAPSULATION - (HIL output)/6(ATS_pHCIDs)
  ATS_pHCIUs_C/1 -> DEVICE ENCAPSULATION - (HIL output)/7(ATS_pHCIUs)
  ATS_pRedAgnt_C/1 -> DEVICE ENCAPSULATION - (HIL output)/8(ATS_pRedAgnt)
  ATS_tHCI_C/1 -> DEVICE ENCAPSULATION - (HIL output)/9(ATS_tHCI)
  ATS_tRedAgntTnk_C/1 -> DEVICE ENCAPSULATION - (HIL output)/12(ATS_tRedAgntTnk)

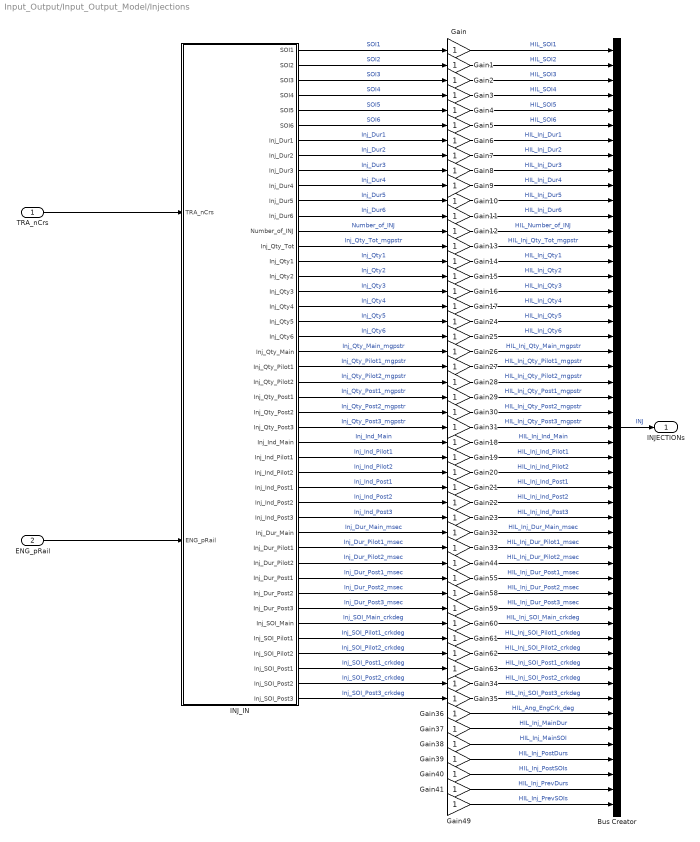
== system Input_Output/Input_Output_Model/Injections ==
  TRA_nCrs : Inport
  ENG_pRail : Inport  Port=2
  Bus Creator : BusCreator  Inputs=51
  Gain{,1..41,44,49,55,58..63} (51 alike) : Gain
  INJ_IN : Subsystem
  INJECTIONs : Outport
  wires:
  Gain49/1 -> Bus Creator/51  "HIL_Inj_PrevSOIs"
  Gain41/1 -> Bus Creator/50  "HIL_Inj_PrevDurs"
  Gain40/1 -> Bus Creator/49  "HIL_Inj_PostSOIs"
  Gain39/1 -> Bus Creator/48  "HIL_Inj_PostDurs"
  Gain38/1 -> Bus Creator/47  "HIL_Inj_MainSOI"
  Gain37/1 -> Bus Creator/46  "HIL_Inj_MainDur"
  Gain35/1 -> Bus Creator/44  "HIL_Inj_SOI_Post3_crkdeg"
  Gain34/1 -> Bus Creator/43  "HIL_Inj_SOI_Post2_crkdeg"
  Gain63/1 -> Bus Creator/42  "HIL_Inj_SOI_Post1_crkdeg"
  Gain62/1 -> Bus Creator/41  "HIL_Inj_SOI_Pilot2_crkdeg"
  Gain61/1 -> Bus Creator/40  "HIL_Inj_SOI_Pilot1_crkdeg"
  Gain60/1 -> Bus Creator/39  "HIL_Inj_SOI_Main_crkdeg"
  Gain59/1 -> Bus Creator/38  "HIL_Inj_Dur_Post3_msec"
  Gain58/1 -> Bus Creator/37  "HIL_Inj_Dur_Post2_msec"
  Gain55/1 -> Bus Creator/36  "HIL_Inj_Dur_Post1_msec"
  Gain44/1 -> Bus Creator/35  "HIL_Inj_Dur_Pilot2_msec"
  Gain33/1 -> Bus Creator/34  "HIL_Inj_Dur_Pilot1_msec"
  Gain32/1 -> Bus Creator/33  "HIL_Inj_Dur_Main_msec"
  Gain23/1 -> Bus Creator/32  "HIL_Inj_Ind_Post3"
  Gain22/1 -> Bus Creator/31  "HIL_Inj_Ind_Post2"
  Gain21/1 -> Bus Creator/30  "HIL_Inj_Ind_Post1"
  Gain20/1 -> Bus Creator/29  "HIL_Inj_Ind_Pilot2"
  Gain19/1 -> Bus Creator/28  "HIL_Inj_Ind_Pilot1"
  Gain18/1 -> Bus Creator/27  "HIL_Inj_Ind_Main"
  Gain31/1 -> Bus Creator/26  "HIL_Inj_Qty_Post3_mgpstr"
  Gain30/1 -> Bus Creator/25  "HIL_Inj_Qty_Post2_mgpstr"
  Gain29/1 -> Bus Creator/24  "HIL_Inj_Qty_Post1_mgpstr"
  Gain28/1 -> Bus Creator/23  "HIL_Inj_Qty_Pilot2_mgpstr"
  Gain27/1 -> Bus Creator/22  "HIL_Inj_Qty_Pilot1_mgpstr"
  Gain26/1 -> Bus Creator/21  "HIL_Inj_Qty_Main_mgpstr"
  Gain25/1 -> Bus Creator/20  "HIL_Inj_Qty6"
  Gain24/1 -> Bus Creator/19  "HIL_Inj_Qty5"
  Gain17/1 -> Bus Creator/18  "HIL_Inj_Qty4"
  Gain16/1 -> Bus Creator/17  "HIL_Inj_Qty3"
  Gain15/1 -> Bus Creator/16  "HIL_Inj_Qty2"
  Gain14/1 -> Bus Creator/15  "HIL_Inj_Qty1"
  Gain13/1 -> Bus Creator/14  "HIL_Inj_Qty_Tot_mgpstr"
  Gain12/1 -> Bus Creator/13  "HIL_Number_of_INJ"
  Gain11/1 -> Bus Creator/12  "HIL_Inj_Dur6"
  Gain10/1 -> Bus Creator/11  "HIL_Inj_Dur5"
  Gain9/1 -> Bus Creator/10  "HIL_Inj_Dur4"
  Gain8/1 -> Bus Creator/9  "HIL_Inj_Dur3"
  Gain7/1 -> Bus Creator/8  "HIL_Inj_Dur2"
  Gain6/1 -> Bus Creator/7  "HIL_Inj_Dur1"
  Gain5/1 -> Bus Creator/6  "HIL_SOI6"
  Gain4/1 -> Bus Creator/5  "HIL_SOI5"
  Gain3/1 -> Bus Creator/4  "HIL_SOI4"
  Gain2/1 -> Bus Creator/3  "HIL_SOI3"
  Gain1/1 -> Bus Creator/2  "HIL_SOI2"
  Gain/1 -> Bus Creator/1  "HIL_SOI1"
  Bus Creator/1 -> INJECTIONs/1  "INJ"
  Gain36/1 -> Bus Creator/45  "HIL_Ang_EngCrk_deg"
  INJ_IN/1(SOI1) -> Gain/1  "SOI1"
  INJ_IN/2(SOI2) -> Gain1/1  "SOI2"
  INJ_IN/3(SOI3) -> Gain2/1  "SOI3"
  INJ_IN/4(SOI4) -> Gain3/1  "SOI4"
  INJ_IN/5(SOI5) -> Gain4/1  "SOI5"
  INJ_IN/6(SOI6) -> Gain5/1  "SOI6"
  INJ_IN/7(Inj_Dur1) -> Gain6/1  "Inj_Dur1"
  INJ_IN/8(Inj_Dur2) -> Gain7/1  "Inj_Dur2"
  INJ_IN/9(Inj_Dur3) -> Gain8/1  "Inj_Dur3"
  INJ_IN/10(Inj_Dur4) -> Gain9/1  "Inj_Dur4"
  INJ_IN/11(Inj_Dur5) -> Gain10/1  "Inj_Dur5"
  INJ_IN/12(Inj_Dur6) -> Gain11/1  "Inj_Dur6"
  INJ_IN/13(Number_of_INJ) -> Gain12/1  "Number_of_INJ"
  INJ_IN/14(Inj_Qty_Tot) -> Gain13/1  "Inj_Qty_Tot_mgpstr"
  INJ_IN/15(Inj_Qty1) -> Gain14/1  "Inj_Qty1"
  INJ_IN/16(Inj_Qty2) -> Gain15/1  "Inj_Qty2"
  INJ_IN/17(Inj_Qty3) -> Gain16/1  "Inj_Qty3"
  INJ_IN/18(Inj_Qty4) -> Gain17/1  "Inj_Qty4"
  INJ_IN/19(Inj_Qty5) -> Gain24/1  "Inj_Qty5"
  INJ_IN/20(Inj_Qty6) -> Gain25/1  "Inj_Qty6"
  INJ_IN/21(Inj_Qty_Main) -> Gain26/1  "Inj_Qty_Main_mgpstr"
  INJ_IN/22(Inj_Qty_Pilot1) -> Gain27/1  "Inj_Qty_Pilot1_mgpstr"
  INJ_IN/23(Inj_Qty_Pilot2) -> Gain28/1  "Inj_Qty_Pilot2_mgpstr"
  INJ_IN/24(Inj_Qty_Post1) -> Gain29/1  "Inj_Qty_Post1_mgpstr"
  INJ_IN/25(Inj_Qty_Post2) -> Gain30/1  "Inj_Qty_Post2_mgpstr"
  INJ_IN/26(Inj_Qty_Post3) -> Gain31/1  "Inj_Qty_Post3_mgpstr"
  INJ_IN/27(Inj_Ind_Main) -> Gain18/1  "Inj_Ind_Main"
  INJ_IN/28(Inj_Ind_Pilot1) -> Gain19/1  "Inj_Ind_Pilot1"
  INJ_IN/29(Inj_Ind_Pilot2) -> Gain20/1  "Inj_Ind_Pilot2"
  INJ_IN/30(Inj_Ind_Post1) -> Gain21/1  "Inj_Ind_Post1"
  INJ_IN/31(Inj_Ind_Post2) -> Gain22/1  "Inj_Ind_Post2"
  INJ_IN/32(Inj_Ind_Post3) -> Gain23/1  "Inj_Ind_Post3"
  INJ_IN/33(Inj_Dur_Main) -> Gain32/1  "Inj_Dur_Main_msec"
  INJ_IN/34(Inj_Dur_Pilot1) -> Gain33/1  "Inj_Dur_Pilot1_msec"
  INJ_IN/35(Inj_Dur_Pilot2) -> Gain44/1  "Inj_Dur_Pilot2_msec"
  INJ_IN/36(Inj_Dur_Post1) -> Gain55/1  "Inj_Dur_Post1_msec"
  INJ_IN/37(Inj_Dur_Post2) -> Gain58/1  "Inj_Dur_Post2_msec"
  INJ_IN/38(Inj_Dur_Post3) -> Gain59/1  "Inj_Dur_Post3_msec"
  INJ_IN/39(Inj_SOI_Main) -> Gain60/1  "Inj_SOI_Main_crkdeg"
  INJ_IN/40(Inj_SOI_Pilot1) -> Gain61/1  "Inj_SOI_Pilot1_crkdeg"
  INJ_IN/41(Inj_SOI_Pilot2) -> Gain62/1  "Inj_SOI_Pilot2_crkdeg"
  INJ_IN/42(Inj_SOI_Post1) -> Gain63/1  "Inj_SOI_Post1_crkdeg"
  INJ_IN/43(Inj_SOI_Post2) -> Gain34/1  "Inj_SOI_Post2_crkdeg"
  INJ_IN/44(Inj_SOI_Post3) -> Gain35/1  "Inj_SOI_Post3_crkdeg"
  ? -> Gain37/1  "Inj_MainDur"
  ? -> Gain38/1  "Inj_MainSOI"
  ? -> Gain39/1  "Inj_PostDurs"
  ? -> Gain40/1  "Inj_PostSOIs"
  ? -> Gain41/1  "Inj_PrevDurs"
  ? -> Gain49/1  "Inj_PrevSOIs"
  TRA_nCrs/1 -> INJ_IN/1(TRA_nCrs)
  ENG_pRail/1 -> INJ_IN/2(ENG_pRail)

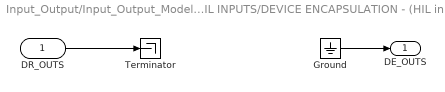
== system Input_Output/Input_Output_Model/HIL INPUTS/DEVICE ENCAPSULATION - (HIL input) ==
  DR_OUTS : Inport
  Ground : Ground
  Terminator : Terminator
  DE_OUTS : Outport
  wires:
  DR_OUTS/1 -> Terminator/1
  Ground/1 -> DE_OUTS/1

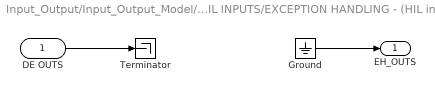
== system Input_Output/Input_Output_Model/HIL INPUTS/EXCEPTION HANDLING - (HIL input) ==
  DE OUTS : Inport
  Ground : Ground
  Terminator : Terminator
  EH_OUTS : Outport
  wires:
  DE OUTS/1 -> Terminator/1
  Ground/1 -> EH_OUTS/1

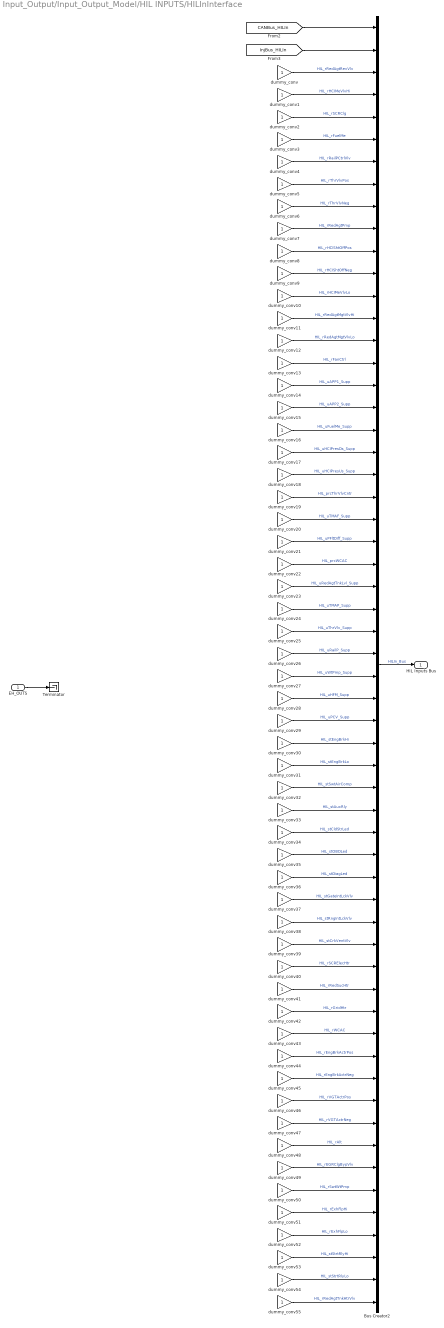
== system Input_Output/Input_Output_Model/HIL INPUTS/HILInInterface ==
  EH_OUTS : Inport
  Bus Creator2 : BusCreator  Inputs=58
  Terminator : Terminator
  dummy_conv{,1..55} (56 alike) : Gain  SaturateOnIntegerOverflow=on  OutDataTypeStr=Inherit: Same as input  ParamDataTypeStr=Inherit: Same as input
  HIL Inputs Bus : Outport
  wires:
  [InjBus_HILIn] -> Bus Creator2/2
  [CANBus_HILIn] -> Bus Creator2/1
  Bus Creator2/1 -> HIL Inputs Bus/1  "HILIn_Bus"
  dummy_conv/1 -> Bus Creator2/3  "HIL_rRedAgtRevVlv"
  dummy_conv1/1 -> Bus Creator2/4  "HIL_rHCIMeVlvHi"
  dummy_conv2/1 -> Bus Creator2/5  "HIL_rSCRClg"
  dummy_conv3/1 -> Bus Creator2/6  "HIL_rFuelMe"
  dummy_conv4/1 -> Bus Creator2/7  "HIL_rRailPCtrlVlv"
  dummy_conv5/1 -> Bus Creator2/8  "HIL_rThrVlvPos"
  dummy_conv6/1 -> Bus Creator2/9  "HIL_rThrVlvNeg"
  dummy_conv7/1 -> Bus Creator2/10  "HIL_rRedAgtPmp"
  dummy_conv8/1 -> Bus Creator2/11  "HIL_rHCIShtOffPos"
  dummy_conv9/1 -> Bus Creator2/12  "HIL_rHCIShtOffNeg"
  dummy_conv10/1 -> Bus Creator2/13  "HIL_rHCIMeVlvLo"
  dummy_conv11/1 -> Bus Creator2/14  "HIL_rRedAgtMgtVlvHi"
  dummy_conv12/1 -> Bus Creator2/15  "HIL_rRedAgtMgtVlvLo"
  dummy_conv13/1 -> Bus Creator2/16  "HIL_rFanCtrl"
  dummy_conv14/1 -> Bus Creator2/17  "HIL_uAPP1_Supp"
  dummy_conv15/1 -> Bus Creator2/18  "HIL_uAPP2_Supp"
  dummy_conv16/1 -> Bus Creator2/19  "HIL_uFuelMe_Supp"
  dummy_conv17/1 -> Bus Creator2/20  "HIL_uHCIPresDs_Supp"
  dummy_conv18/1 -> Bus Creator2/21  "HIL_uHCIPresUs_Supp"
  dummy_conv19/1 -> Bus Creator2/22  "HIL_prcThrVlvCntr"
  dummy_conv20/1 -> Bus Creator2/23  "HIL_uTMAF_Supp"
  dummy_conv21/1 -> Bus Creator2/24  "HIL_uPFltDiff_Supp"
  dummy_conv22/1 -> Bus Creator2/25  "HIL_prcWCAC"
  dummy_conv23/1 -> Bus Creator2/26  "HIL_uRedAgtTnkLvl_Supp"
  dummy_conv24/1 -> Bus Creator2/27  "HIL_uTMAP_Supp"
  dummy_conv25/1 -> Bus Creator2/28  "HIL_uThrVlv_Supp"
  dummy_conv26/1 -> Bus Creator2/29  "HIL_uRailP_Supp"
  dummy_conv27/1 -> Bus Creator2/30  "HIL_uWtPmp_Supp"
  dummy_conv28/1 -> Bus Creator2/31  "HIL_uHFM_Supp"
  dummy_conv29/1 -> Bus Creator2/32  "HIL_uPCV_Supp"
  dummy_conv30/1 -> Bus Creator2/33  "HIL_stEngBrkHi"
  dummy_conv31/1 -> Bus Creator2/34  "HIL_stEngBrkLo"
  dummy_conv32/1 -> Bus Creator2/35  "HIL_stSwtAirComp"
  dummy_conv33/1 -> Bus Creator2/36  "HIL_stAuxRly"
  dummy_conv34/1 -> Bus Creator2/37  "HIL_stCldStrLed"
  dummy_conv35/1 -> Bus Creator2/38  "HIL_stOBDLed"
  dummy_conv36/1 -> Bus Creator2/39  "HIL_stDiagLed"
  dummy_conv37/1 -> Bus Creator2/40  "HIL_stGateIntLckVlv"
  dummy_conv38/1 -> Bus Creator2/41  "HIL_stRngIntLckVlv"
  dummy_conv39/1 -> Bus Creator2/42  "HIL_stCrkVentVlv"
  dummy_conv40/1 -> Bus Creator2/43  "HIL_rSCRElecHtr"
  dummy_conv41/1 -> Bus Creator2/44  "HIL_rRedSucHtr"
  dummy_conv42/1 -> Bus Creator2/45  "HIL_rGridHtr"
  dummy_conv43/1 -> Bus Creator2/46  "HIL_rWCAC"
  dummy_conv44/1 -> Bus Creator2/47  "HIL_rEngBrkActrPos"
  dummy_conv45/1 -> Bus Creator2/48  "HIL_rEngBrkActrNeg"
  dummy_conv46/1 -> Bus Creator2/49  "HIL_rVGTActrPos"
  dummy_conv47/1 -> Bus Creator2/50  "HIL_rVGTActrNeg"
  dummy_conv48/1 -> Bus Creator2/51  "HIL_rAlt"
  dummy_conv49/1 -> Bus Creator2/52  "HIL_rEGRClgBypVlv"
  dummy_conv50/1 -> Bus Creator2/53  "HIL_rSwtWtPmp"
  dummy_conv51/1 -> Bus Creator2/54  "HIL_rExhFlpHi"
  dummy_conv52/1 -> Bus Creator2/55  "HIL_rExhFlpLo"
  dummy_conv53/1 -> Bus Creator2/56  "HIL_stStrtRlyHi"
  dummy_conv54/1 -> Bus Creator2/57  "HIL_stStrtRlyLo"
  dummy_conv55/1 -> Bus Creator2/58  "HIL_rRedAgtTnkHtrVlv"
  EH_OUTS/1 -> Terminator/1

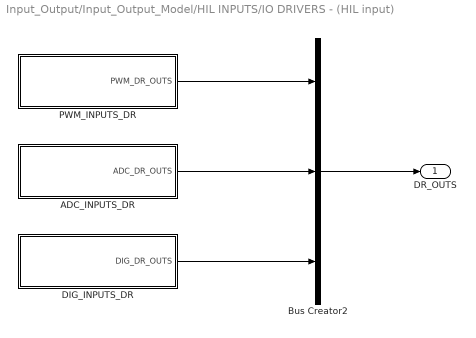
== system Input_Output/Input_Output_Model/HIL INPUTS/IO DRIVERS - (HIL input) ==
  ADC_INPUTS_DR : Subsystem
  Bus Creator2 : BusCreator  Inputs=3
  DIG_INPUTS_DR : Subsystem
  PWM_INPUTS_DR : Subsystem
  DR_OUTS : Outport
  wires:
  Bus Creator2/1 -> DR_OUTS/1
  DIG_INPUTS_DR/1("DIG_DR_OUTS ") -> Bus Creator2/3
  ADC_INPUTS_DR/1("ADC_DR_OUTS ") -> Bus Creator2/2
  PWM_INPUTS_DR/1("PWM_DR_OUTS ") -> Bus Creator2/1

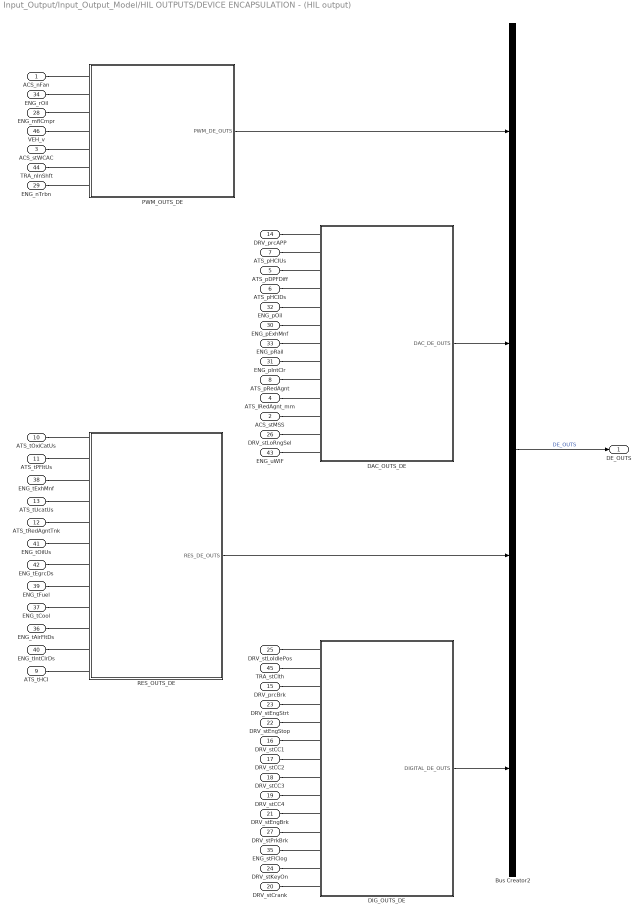
== system Input_Output/Input_Output_Model/HIL OUTPUTS/DEVICE ENCAPSULATION - (HIL output) ==
  ACS_nFan : Inport
  ACS_stMSS : Inport  Port=2
  ACS_stWCAC : Inport  Port=3
  ATS_lRedAgnt_mm : Inport  Port=4
  ATS_pDPFDiff : Inport  Port=5
  ATS_pHCIDs : Inport  Port=6
  ATS_pHCIUs : Inport  Port=7
  ATS_pRedAgnt : Inport  Port=8
  ATS_tHCI : Inport  Port=9
  ATS_tOxiCatUs : Inport  Port=10
  ATS_tPFltUs : Inport  Port=11
  ATS_tRedAgntTnk : Inport  Port=12
  ATS_tUcatUs : Inport  Port=13
  DRV_prcAPP : Inport  Port=14
  DRV_prcBrk : Inport  Port=15
  DRV_stCC1 : Inport  Port=16
  DRV_stCC2 : Inport  Port=17
  DRV_stCC3 : Inport  Port=18
  DRV_stCC4 : Inport  Port=19
  DRV_stCrank : Inport  Port=20
  DRV_stEngBrk : Inport  Port=21
  DRV_stEngStop : Inport  Port=22
  DRV_stEngStrt : Inport  Port=23
  DRV_stKeyOn : Inport  Port=24
  DRV_stLoIdlePos : Inport  Port=25
  DRV_stLoRngSel : Inport  Port=26
  DRV_stPrkBrk : Inport  Port=27
  ENG_mflCmpr : Inport  Port=28
  ENG_nTrbn : Inport  Port=29
  ENG_pExhMnf : Inport  Port=30
  ENG_pIntClr : Inport  Port=31
  ENG_pOil : Inport  Port=32
  ENG_pRail : Inport  Port=33
  ENG_rOil : Inport  Port=34
  ENG_stFlClog : Inport  Port=35
  ENG_tAirFltDs : Inport  Port=36
  ENG_tCool : Inport  Port=37
  ENG_tExhMnf : Inport  Port=38
  ENG_tFuel : Inport  Port=39
  ENG_tIntClrDs : Inport  Port=40
  ENG_tOilUs : Inport  Port=41
  ENG_tEgrcDs : Inport  Port=42
  ENG_uWIF : Inport  Port=43
  TRA_nInShft : Inport  Port=44
  TRA_stClth : Inport  Port=45
  VEH_v : Inport  Port=46
  Bus Creator2 : BusCreator  Inputs=4
  DAC_OUTS_DE : Subsystem
  DIG_OUTS_DE : Subsystem
  PWM_OUTS_DE : Subsystem
  RES_OUTS_DE : Subsystem
  DE_OUTS : Outport
  wires:
  DIG_OUTS_DE/1(DIGITAL_DE_OUTS) -> Bus Creator2/4
  RES_OUTS_DE/1(RES_DE_OUTS) -> Bus Creator2/3
  Bus Creator2/1 -> DE_OUTS/1  "DE_OUTS"
  PWM_OUTS_DE/1(PWM_DE_OUTS) -> Bus Creator2/1
  DAC_OUTS_DE/1(DAC_DE_OUTS) -> Bus Creator2/2
  ACS_nFan/1 -> ?
  ENG_rOil/1 -> ?
  ENG_mflCmpr/1 -> ?
  VEH_v/1 -> ?
  ACS_stWCAC/1 -> ?
  TRA_nInShft/1 -> ?
  ENG_nTrbn/1 -> ?
  ATS_pHCIDs/1 -> ?
  ATS_pDPFDiff/1 -> ?
  ENG_pOil/1 -> ?
  ATS_pHCIUs/1 -> ?
  ENG_pExhMnf/1 -> ?
  DRV_prcAPP/1 -> ?
  ENG_pRail/1 -> ?
  ENG_pIntClr/1 -> ?
  ATS_pRedAgnt/1 -> ?
  ATS_lRedAgnt_mm/1 -> ?
  ACS_stMSS/1 -> ?
  DRV_stLoRngSel/1 -> ?
  ENG_uWIF/1 -> ?
  ATS_tOxiCatUs/1 -> ?
  ATS_tHCI/1 -> ?
  ATS_tPFltUs/1 -> ?
  ENG_tExhMnf/1 -> ?
  ENG_tFuel/1 -> ?
  ENG_tCool/1 -> ?
  ENG_tAirFltDs/1 -> ?
  ENG_tIntClrDs/1 -> ?
  ENG_tEgrcDs/1 -> ?
  ENG_tOilUs/1 -> ?
  ATS_tUcatUs/1 -> ?
  ATS_tRedAgntTnk/1 -> ?
  DRV_stLoIdlePos/1 -> ?
  TRA_stClth/1 -> ?
  DRV_prcBrk/1 -> ?
  DRV_stEngStrt/1 -> ?
  DRV_stEngStop/1 -> ?
  DRV_stCC1/1 -> ?
  DRV_stCC2/1 -> ?
  DRV_stCC3/1 -> ?
  DRV_stCC4/1 -> ?
  DRV_stEngBrk/1 -> ?
  DRV_stPrkBrk/1 -> ?
  ENG_stFlClog/1 -> ?
  DRV_stKeyOn/1 -> ?
  DRV_stCrank/1 -> ?

== system Input_Output/Input_Output_Model/HIL OUTPUTS/EXCEPTION HANDLING - (HIL output) ==
  DE_OUTS : Inport
  Ground : Ground
  Terminator : Terminator
  EH_OUTS : Outport
  wires:
  DE_OUTS/1 -> Terminator/1
  Ground/1 -> EH_OUTS/1

== system Input_Output/Input_Output_Model/HIL OUTPUTS/IO DRIVERS - (HIL output) ==
  EH_OUTS : Inport
  Terminator : Terminator
  wires:
  EH_OUTS/1 -> Terminator/1

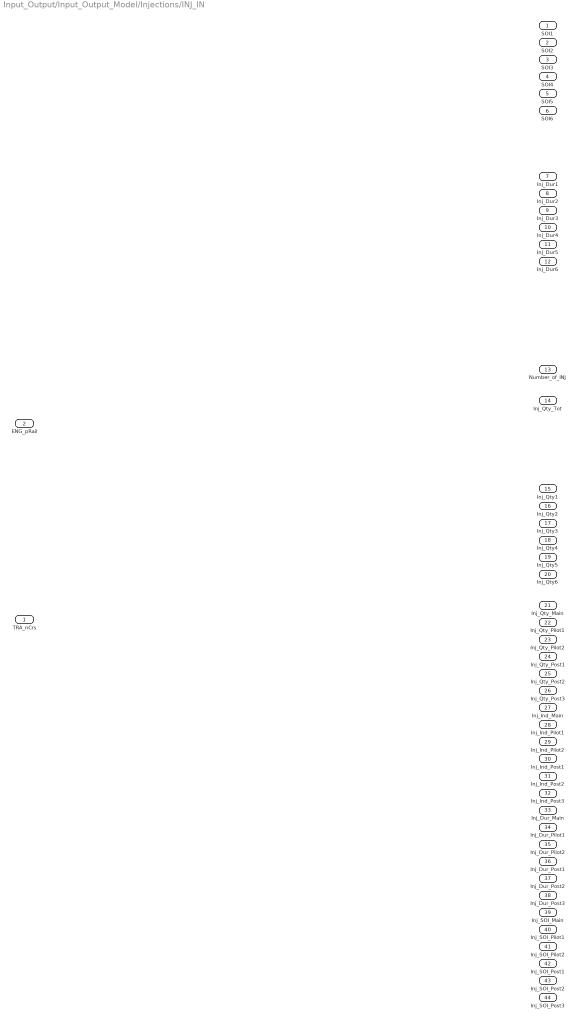
== system Input_Output/Input_Output_Model/Injections/INJ_IN ==
  TRA_nCrs : Inport
  ENG_pRail : Inport  Port=2
  SOI1 : Outport
  SOI2 : Outport  Port=2
  SOI3 : Outport  Port=3
  SOI4 : Outport  Port=4
  SOI5 : Outport  Port=5
  SOI6 : Outport  Port=6
  Inj_Dur1 : Outport  Port=7
  Inj_Dur2 : Outport  Port=8
  Inj_Dur3 : Outport  Port=9
  Inj_Dur4 : Outport  Port=10
  Inj_Dur5 : Outport  Port=11
  Inj_Dur6 : Outport  Port=12
  Number_of_INJ : Outport  Port=13
  Inj_Qty_Tot : Outport  Port=14
  Inj_Qty1 : Outport  Port=15
  Inj_Qty2 : Outport  Port=16
  Inj_Qty3 : Outport  Port=17
  Inj_Qty4 : Outport  Port=18
  Inj_Qty5 : Outport  Port=19
  Inj_Qty6 : Outport  Port=20
  Inj_Qty_Main : Outport  Port=21
  Inj_Qty_Pilot1 : Outport  Port=22
  Inj_Qty_Pilot2 : Outport  Port=23
  Inj_Qty_Post1 : Outport  Port=24
  Inj_Qty_Post2 : Outport  Port=25
  Inj_Qty_Post3 : Outport  Port=26
  Inj_Ind_Main : Outport  Port=27
  Inj_Ind_Pilot1 : Outport  Port=28
  Inj_Ind_Pilot2 : Outport  Port=29
  Inj_Ind_Post1 : Outport  Port=30
  Inj_Ind_Post2 : Outport  Port=31
  Inj_Ind_Post3 : Outport  Port=32
  Inj_Dur_Main : Outport  Port=33
  Inj_Dur_Pilot1 : Outport  Port=34
  Inj_Dur_Pilot2 : Outport  Port=35
  Inj_Dur_Post1 : Outport  Port=36
  Inj_Dur_Post2 : Outport  Port=37
  Inj_Dur_Post3 : Outport  Port=38
  Inj_SOI_Main : Outport  Port=39
  Inj_SOI_Pilot1 : Outport  Port=40
  Inj_SOI_Pilot2 : Outport  Port=41
  Inj_SOI_Post1 : Outport  Port=42
  Inj_SOI_Post2 : Outport  Port=43
  Inj_SOI_Post3 : Outport  Port=44

== system Input_Output/Input_Output_Model/HIL INPUTS/IO DRIVERS - (HIL input)/ADC_INPUTS_DR ==
  Bus Creator1 : BusCreator  Inputs=16
  "ADC_DR_OUTS " : Outport
  wires:
  Bus Creator1/1 -> "ADC_DR_OUTS "/1  "ADC_DR_OUTS"

== system Input_Output/Input_Output_Model/HIL INPUTS/IO DRIVERS - (HIL input)/DIG_INPUTS_DR ==
  Bus Creator2 : BusCreator  Inputs=26
  "DIG_DR_OUTS " : Outport
  wires:
  Bus Creator2/1 -> "DIG_DR_OUTS "/1  "DIG_DR_OUTS"

== system Input_Output/Input_Output_Model/HIL INPUTS/IO DRIVERS - (HIL input)/PWM_INPUTS_DR ==
  Bus Creator2 : BusCreator  Inputs=14
  "PWM_DR_OUTS " : Outport
  wires:
  Bus Creator2/1 -> "PWM_DR_OUTS "/1  "PWM_DR_OUTS"

== system Input_Output/Input_Output_Model/HIL OUTPUTS/DEVICE ENCAPSULATION - (HIL output)/DAC_OUTS_DE ==
  Bus Creator2 : BusCreator  Inputs=14
  DAC_DE_OUTS : Outport
  wires:
  Bus Creator2/1 -> DAC_DE_OUTS/1  "DAC_DE_OUTS"

== system Input_Output/Input_Output_Model/HIL OUTPUTS/DEVICE ENCAPSULATION - (HIL output)/DIG_OUTS_DE ==
  Bus Creator1 : BusCreator  Inputs=15
  DIGITAL_DE_OUTS : Outport
  wires:
  Bus Creator1/1 -> DIGITAL_DE_OUTS/1  "DIG_DE_OUTS"

== system Input_Output/Input_Output_Model/HIL OUTPUTS/DEVICE ENCAPSULATION - (HIL output)/PWM_OUTS_DE ==
  Bus Creator2 : BusCreator  Inputs=7
  PWM_DE_OUTS : Outport
  wires:
  Bus Creator2/1 -> PWM_DE_OUTS/1  "PWM_DE_OUTS"

== system Input_Output/Input_Output_Model/HIL OUTPUTS/DEVICE ENCAPSULATION - (HIL output)/RES_OUTS_DE ==
  Bus Creator1 : BusCreator  Inputs=12
  RES_DE_OUTS : Outport
  wires:
  Bus Creator1/1 -> RES_DE_OUTS/1  "RES_DE_OUTS"
